simulink model "hydraulic_pilot_dashboard_US"  (R2015b)
settings: Solver=ode23t  StartTime=0.0  StopTime=1500  RelTol=1e-3
undefined symbols (not defined in the file): X, Y, Z
libraries: sm_lib x295, fl_lib x24, nesl_utility x13, sh_lib x5, simulink x1
(part 1 of 7)
settings Model: Creator=Ivan  LastModifiedBy=Ivan
settings DataIOCC: SaveFormat=Array
settings DebuggingCC: UnderspecifiedInitializationDetection=Classic  MergeDetectMultiDrivingBlocksExec=none  SolverPrmCheckMsg=warning  StateNameClashWarn=warning
settings HardwareCC: ProdBitPerPointer=32  ProdLargestAtomicFloat=None  ProdIntDivRoundTo=Undefined  ProdEndianess=Unspecified  ProdWordSize=32  ProdHWDeviceType=32-bit Generic
settings GRTTargetCC: GeneratePreprocessorConditionals=Disable all
settings ConfigComp: CovModelRefEnable=Off
settings SimscapeCC: SimscapeLogType=all  SimscapeLogLimitData=off
settings ExplorerConfigSet: InternalSimMechanicsExplorerSettings="<ExplorerConfiguration><canonicalview>default</canonicalview><AnimationSetting><BasePlaybackSpeed>1.0</BasePlaybackSpeed><PlaybackSpeedFactor>16.0</PlaybackSpeedFactor></AnimationSetting><TilePanel><TileInfo><Tiles Columns=\"2\" Count=\"4\" Rows=\"2\"><Column Left=\"2\" Weight=\"0.5\"/><Column Left=\"554\" Weight=\"0.5\"/><Column Left=\"1106\"/><Row Top=\"2\" Weight=\"0.4992\"/><Row Top=\"320\" Weight=\"0.5008\"/><Row Top=\"639\"/><Tile Height=\"1\" Width=\"1\" X=\"0\" Y=\"0\"/><Tile Height=\"1\" Width=\"1\" X=\"0\" Y=\"1\"/><Tile Height=\"1\" Width=\"1\" X=\"1\" Y=\"0\"/><Tile Height=\"1\" Width=\"1\" X=\"1\" Y=\"1\"/></Tiles></TileInfo><SceneInfo><SceneViewer><BGColor><R>0.60000002384185791</R><G>0.60000002384185791</G><B>0.60000002384185791</B></BGColor><Camera><Position><X>-1.4545420789578025</X><Y>-0.47703526853152423</Y><Z>1.053292472596125</Z></Position><Center><X>-1.0755331343287176</X><Y>0.65681441625729753</Y><Z>0.33046154790126991</Z></Center><Up><X>0.31799715127972389</X><Y>0.43179203595848165</Y><Z>0.84405772874893448</Z></Up><Left>-0.52137946486473086</Left><Right>0.52137946486473086</Right><Bottom>-0.12744375988841058</Bottom><Top>0.12744375988841058</Top></Camera></SceneViewer><SceneViewer><BGColor><R>0.60000002384185791</R><G>0.60000002384185791</G><B>0.60000002384185791</B></BGColor><Camera><Position><X>-1.097124655307177</X><Y>0.60879350298107193</Y><Z>1.6773847746848054</Z></Position><Center><X>-1.097124655307177</X><Y>0.60879350298107193</Y><Z>0.3230140209197998</Z></Center><Up><X>0</X><Y>1</Y><Z>-0</Z></Up><Left>-0.52137946486473086</Left><Right>0.52137946486473086</Right><Bottom>-0.19162502065300943</Bottom><Top>0.19162502065300943</Top></Camera></SceneViewer><SceneViewer><BGColor><R>0.60000002384185791</R><G>0.60000002384185791</G><B>0.60000002384185791</B></BGColor><Camera><Position><X>-1.839713975613805</X><Y>1.4497817237667032</Y><Z>1.0667372871108483</Z></Position><Center><X>-1.0007040048852538</X><Y>0.55541256489420043</Y><Z>0.26430212739881542</Z></Center><Up><X>0.29701754457873719</X><Y>-0.46808723288325788</Y><Z>0.83227094183571793</Z></Up><Left>-0.47525307471029621</Left><Right>0.47525307471029621</Right><Bottom>-0.31607583672115108</Bottom><Top>0.31607583672115108</Top></Camera></SceneViewer><SceneViewer><BGColor><R>0.60000002384185791</R><G>0.60000002384185791</G><B>0.60000002384185791</B></BGColor><Camera><Position><X>-0.30663977538297038</X><Y>-0.17371608341982503</Y><Z>1.1012231263046517</Z></Position><Center><X>-1.0848488807678223</X><Y>0.60449302196502686</Y><Z>0.3230140209197998</Z></Center><Up><X>-0.40824829046386307</X><Y>0.40824829046386307</Y><Z>0.81649658092772615</Z></Up><Left>-0.50417031347751617</Left><Right>0.50417031347751617</Right><Bottom>-0.39514026045799255</Bottom><Top>0.39514026045799255</Top></Camera></SceneViewer></SceneInfo></TilePanel></ExplorerConfiguration>"

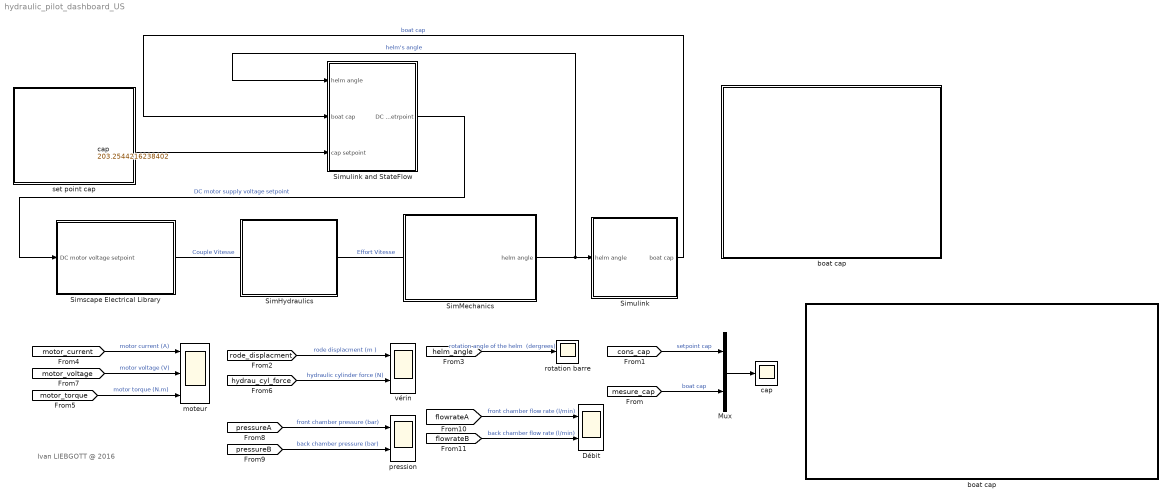
== system hydraulic_pilot_dashboard_US ==
  note: Ivan LIEBGOTT @ 2016
  " moteur" : Scope  NumInputPorts=3
  Débit : Scope  NumInputPorts=2
  Mux : Mux  Inputs=2
  SimHydraulics : Subsystem
      mask Display: image('groupe_hydraulique.jpg')
  SimMechanics : Subsystem
      mask Display: image('pilote_simmechanics.jpg')
  "Simscape Electrical Library " : Subsystem
      mask Display: image('moteur_cc_pilote.jpg')
  Simulink : Subsystem
      mask Display: image('bateau.jpg')
  Simulink and StateFlow : Subsystem
      mask Display: image('AP16_FRONT.jpg')
  boat cap : Subsystem  DialogController=hmiCreateDDGDialog  IsWebBlock=on  mask(MathWorksWebBlock){webBlockId=e22fa1aa-ddbe-4e38-8835-48dbfeb78bab, webBlockType=sdiscope, ShowInitialText=on, HMISrcModelName=hydraulic_pilot_dashboard_US}
      mask prompts: webBlockId "WebBlock Id"; webBlockType "WebBlock Type"; HMISrcModelName "Source Model"
      mask Help: helpview([docroot '/mapfiles/simulink.map'], 'hmi_scope')
      mask Display:
      | if strcmp(get_param(bdroot(gcb),'BlockDiagramType'), 'library')
      |     image([(matlabroot) '/toolbox/simulink/hmi/icons/DashboardScope.png']);
      | end
  "boat cap " : Subsystem  DialogController=hmiCreateDDGDialog  IsWebBlock=on  mask(MathWorksWebBlock){webBlockId=00e2b6f1-632d-4b1a-952e-7d57ffc56f45, webBlockType=circulargauge, ShowInLibBrowser=on, ShowInitialText=on, HMISrcModelName=hydraulic_pilot_dashboard_US}
      mask prompts: webBlockId "WebBlock Id"; webBlockType "WebBlock Type"; HMISrcModelName "Source Model"
      mask Help: helpview([docroot '/mapfiles/simulink.map'], 'hmi_gauge')
      mask Display:
      | if strcmp(get_param(bdroot(gcb),'BlockDiagramType'), 'library')
      |     image([(matlabroot) '/toolbox/simulink/hmi/icons/CircularGauge.png']);
      | end
  cap : Constant  Value=203.2544216238402
  "cap " : Scope
  pression : Scope  NumInputPorts=2
  rotation barre : Scope
  set point cap : Subsystem  DialogController=hmiCreateDDGDialog  IsWebBlock=on  mask(MathWorksWebBlock){webBlockId=deb2e274-1bba-45a5-ab0e-2b4103336ddf, webBlockType=continuousknob, ShowInLibBrowser=on, ShowInitialText=on, HMISrcModelName=hydraulic_pilot_dashboard_US}
      mask prompts: webBlockId "WebBlock Id"; webBlockType "WebBlock Type"; HMISrcModelName "Source Model"
      mask Help: helpview([docroot '/mapfiles/simulink.map'], 'hmi_knob')
      mask Display:
      | if strcmp(get_param(bdroot(gcb),'BlockDiagramType'), 'library')
      |     image([(matlabroot) '/toolbox/simulink/hmi/icons/ContinuousKnob.png']);
      | end
  vérin : Scope  NumInputPorts=2
  wires:
  SimMechanics/1(helm angle) -> Simulink/1(helm angle), Simulink and StateFlow/1(helm angle)  "helm's angle"
  Mux/1 -> "cap "/1
  [mesure_cap] -> Mux/2  "boat cap"
  [cons_cap] -> Mux/1  "setpoint cap"
  [rode_displacment] -> vérin/1  "rode displacment (m )"
  [helm_angle] -> rotation barre/1  "rotation angle of the helm  (dergrees)"
  [motor_current] -> " moteur"/1  "motor current (A)"
  [motor_torque] -> " moteur"/3  "motor torque (N.m)"
  [hydrau_cyl_force] -> vérin/2  "hydraulic cylinder force (N)"
  cap/1 -> Simulink and StateFlow/3(cap setpoint)
  Simulink/1(boat cap) -> Simulink and StateFlow/2(boat cap)  "boat cap"
  Simulink and StateFlow/1(DC motor voltage setrpoint) -> "Simscape Electrical Library "/1(DC motor voltage setpoint)  "DC motor supply voltage setpoint"
  [motor_voltage] -> " moteur"/2  "motor voltage (V)"
  [pressureA] -> pression/1  "front chamber pressure (bar)"
  [pressureB] -> pression/2  "back chamber pressure (bar)"
  [flowrateA] -> Débit/1  "front chamber flow rate (l/min)"
  [flowrateB] -> Débit/2  "back chamber flow rate (l/min)"
  connections:
  "Simscape Electrical Library "/RConn1 -- SimHydraulics/LConn1  "Couple Vitesse"
  SimHydraulics/RConn1 -- SimMechanics/LConn1  "Effort Vitesse"

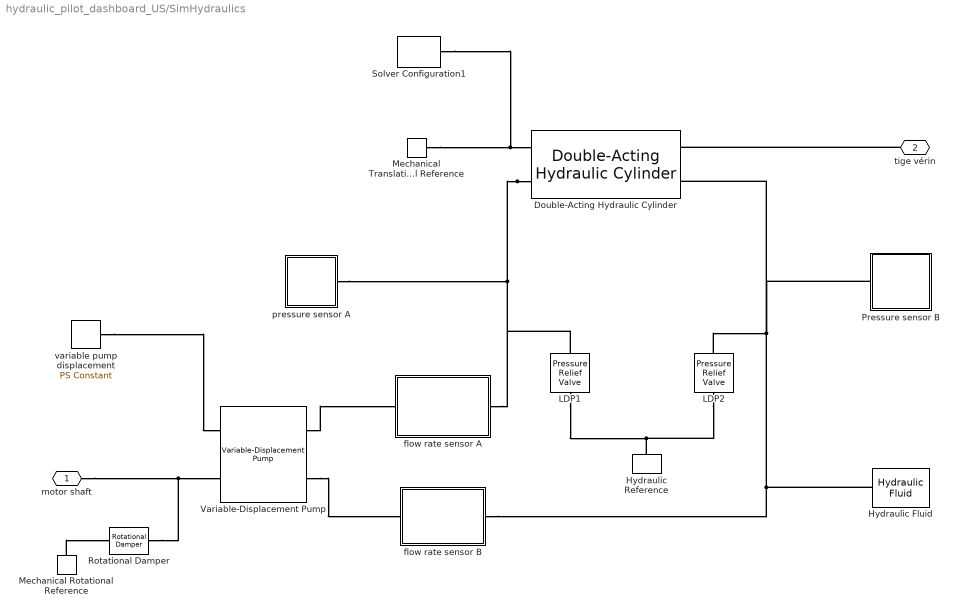
== system hydraulic_pilot_dashboard_US/SimHydraulics ==
  " LDP1" : sh_lib/Valves/Pressure Control Valves/Pressure Relief Valve  area_max=1e-4 m^2  pres_set=10e+6 Pa  reg_range=5e+5 Pa  C_d=0.7  Re_cr=12  A_leak=1e-12 m^2  dynamic=0  tau=0.1 s  area_init=1e-12 m^2  gain=1 m^2/Pa  pr_max=55e5 Pa  f_cr=100 N
  Double-Acting Hydraulic Cylinder : sh_lib/Hydraulic Cylinders/Double-Acting Hydraulic Cylinder  area_A=2e-4 m^2  area_B=2e-4 m^2  stroke=0.3 m  init_pos=0.15 m  dead_vol_A=1e-4 m^3  dead_vol_B=1e-4 m^3  init_pressure_A=0 Pa  init_pressure_B=0 Pa  k_sh=1.4  stiff=1e+6 N/m  D=150 N/(m/s)  or=1  or_sign=1
  Hydraulic Fluid : sh_lib/Hydraulic Utilities/Hydraulic Fluid  DataSource=1  SelFluid=1  SysTemp=60 c  TrapAir=0.005  ViscDerFactor=1  range_error=2
  Hydraulic Reference : fl_lib/Hydraulic/Hydraulic Elements/Hydraulic Reference
  LDP2 : sh_lib/Valves/Pressure Control Valves/Pressure Relief Valve  area_max=1e-4 m^2  pres_set=10e+6 Pa  reg_range=5e+5 Pa  C_d=0.7  Re_cr=12  A_leak=1e-12 m^2  dynamic=0  tau=0.1 s  area_init=1e-12 m^2  gain=1 m^2/Pa  pr_max=55e5 Pa  f_cr=100 N
  Mechanical Rotational Reference : fl_lib/Mechanical/Rotational Elements/Mechanical Rotational Reference
  Mechanical Translational Reference : fl_lib/Mechanical/Translational Elements/Mechanical Translational Reference
  Pressure sensor B : Subsystem
      mask Display: image('manometre.jpg')
  Rotational Damper : fl_lib/Mechanical/Rotational Elements/Rotational Damper  D=0.006 N*m/(rad/s)  w_specify=off  w_priority=None  w=0 rad/s  t_specify=off  t_priority=None  t=0 N*m
  Solver Configuration1 : nesl_utility/Solver Configuration  PhysicalDomain=network_engine_domain  SubClassName=solver  LeftPortType=input  RightPortType=generic  Accelerate=off  Tones=[]  Harmonics=[]  SimulateNoise=off  Profile=off  UseLocalSampling=off  EnableSwitchedLinearOptims=on  FrequencyDomain=off  UseCCode=off  RelTol=0.001  AbsTol=1e-06  MinStep=1e-09  ToWorkspace=off  RevertToSquareIcSolve=off  NumHomotopyIterations=100  PhasorMode=off  PhasorModeNumHarmonics=1  DoDC=off  ResidualTolerance=1e-09  UseLocalSolver=off  LocalSolverChoice=NE_BACKWARD_EULER_ADVANCER  LocalSolverSampleTime=0.001  DoFixedCost=off  MaxNonlinIter=3  MaxModeIter=2  LinearAlgebra=Sparse  DelaysMemoryBudget=1024  AutomaticFiltering=on  FilteringTimeConstant=0.001
  Variable-Displacement Pump : sh_lib/Pumps and Motors/Variable-Displacement Pump  mdl_type=1  D_max=1.77e-7 m^3/rad  stroke_max=1 m  displ_tab=[ -5e-6 -3e-6 0 3e-6 5e-6 ] m^3/rad  cntrl_mem_tab=[ -0.0075 -0.0025 0 0.0025 0.0075 ] m  interp_method=1  extrap_method=1  efficiency_vol=0.85  efficiency_tot=0.75  pr_nominal=1e+8 Pa  w_nominal=188 rad/s  visc_nominal=18 cSt  dens_nominal=900 kg/m^3  k_leak=1e-11 m^3/s/Pa  efficiency_mech=0.7
  flow rate sensor A : Subsystem
      mask Display: image('debimetre.jpg')
  flow rate sensor B : Subsystem
      mask Display: image('debimetre.jpg')
  pressure sensor A : Subsystem
      mask Display: image('manometre.jpg')
  variable pump displacement : fl_lib/Physical Signals/Sources/PS Constant  constant=0.4
  motor shaft : PMIOPort  Port=1  Side=Left
  tige vérin : PMIOPort  Port=2  Side=Right
  connections:
  motor shaft/RConn1 -- Rotational Damper/RConn1 -- Variable-Displacement Pump/LConn2
  variable pump displacement/RConn1 -- Variable-Displacement Pump/LConn1
  tige vérin/RConn1 -- Double-Acting Hydraulic Cylinder/RConn1
  Mechanical Translational Reference/LConn1 -- Solver Configuration1/RConn1 -- Double-Acting Hydraulic Cylinder/LConn1
  Hydraulic Fluid/RConn1 -- flow rate sensor B/RConn1 -- Pressure sensor B/LConn1 -- Double-Acting Hydraulic Cylinder/RConn2 -- LDP2/LConn1
  Hydraulic Reference/LConn1 -- " LDP1"/RConn1 -- LDP2/RConn1
  Mechanical Rotational Reference/LConn1 -- Rotational Damper/LConn1
  Double-Acting Hydraulic Cylinder/LConn2 -- flow rate sensor A/RConn1 -- " LDP1"/LConn1 -- pressure sensor A/RConn1
  Variable-Displacement Pump/RConn1 -- flow rate sensor A/LConn1
  Variable-Displacement Pump/RConn2 -- flow rate sensor B/LConn1

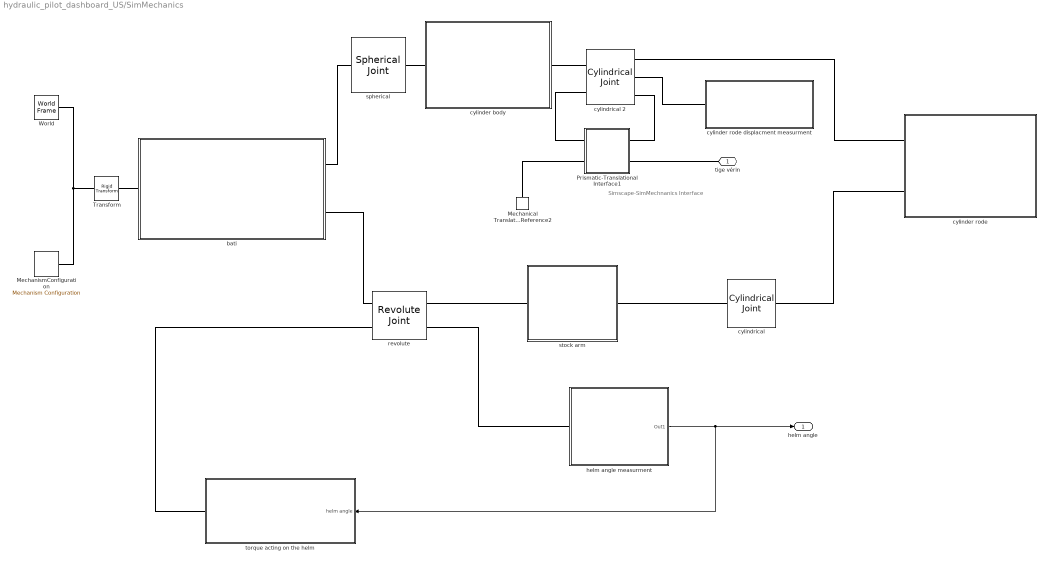
== system hydraulic_pilot_dashboard_US/SimMechanics ==
  note: Simscape-SimMechnanics
      |  Interface
  Mechanical Translational Reference2 : fl_lib/Mechanical/Translational Elements/Mechanical Translational Reference
  MechanismConfiguration : sm_lib/Utilities/Mechanism Configuration  UniformGravity=Constant  GravityVector=[0 0 -9.81]  GravityUnits=m/s^2  LinearizationDelta=0.001  BlockFunction=simmechanics.library.utilities.mechanism_configuration
  Prismatic-Translational Interface1 : Subsystem
  Transform : sm_lib/Frames and Transforms/Rigid Transform  TranslationMethod=Cartesian  TranslationLengthUnit=mm  TranslationStandardAxis=+Z  TranslationStandardOffset=0  TranslationCartesianOffset=[-854.29700000000003 517.99300000000005 336.38900000000001]  TranslationROffset=0  TranslationROffsetUnits=m  TranslationZOffset=0  TranslationZOffsetUnits=m  TranslationThetaOffset=0  TranslationThetaOffsetUnits=deg  RotationMethod=None  RotationAngleUnits=deg  RotationStandardAxis=+Z  RotationAngle=0  RotationArbitraryAxis=[0 0 1]  FollAlignAxisA=+X  BaseAlignAxisA=+Y  FollAlignAxisB=+Y  BaseAlignAxisB=+Z  RotationSequenceAxes=FollowerAxes  RotationSequence=XYX  RotationSequenceAngles=[0 0 0]  RotationSequenceAnglesUnits=deg  RotationMatrix=[1 0 0; 0 1 0; 0 0 1]  BlockFunction=simmechanics.library.frames_transforms.rigid_transform
  World : sm_lib/Frames and Transforms/World Frame  BlockFunction=simmechanics.library.frames_transforms.world_frame
  bati : Subsystem
      mask Display: image('bati1.jpg')
  cylinder body : Subsystem
      mask Display: image('cylindre.jpg')
  cylinder rode : Subsystem
      mask Display: image('tige1.jpg')
  cylinder rode displacment measurment : Subsystem
      mask Display: image('potentiometrelineaire.jpg')
  cylindrical : sm_lib/Joints/Cylindrical Joint  SenseConstraintForce=off  SenseConstraintForceX=off  SenseConstraintForceY=off  SenseConstraintForceZ=off  SenseConstraintTorque=off  SenseConstraintTorqueX=off  SenseConstraintTorqueY=off  SenseConstraintTorqueZ=off  SenseTotalForce=off  SenseTotalForceX=off  SenseTotalForceY=off  SenseTotalForceZ=off  SenseTotalTorque=off  SenseTotalTorqueX=off  SenseTotalTorqueY=off  SenseTotalTorqueZ=off  CompositeWrenchDir=FollowerOnBase  CompositeWrenchFrame=BaseFrame  PzEquilibriumPosition=0  PzEquilibriumPositionUnits=m  PzSpringStiffness=0  PzSpringStiffnessUnits=N/m  PzDampingCoefficient=0  PzDampingCoefficientUnits=s*N/m  PzTorqueActuationMode=NoTorque  PzMotionActuationMode=ComputedMotion  PzSensePosition=off  PzSenseVelocity=off  PzSenseAcceleration=off  PzSenseTorqueForce=off  PzPositionTargetSpecify=on  PzPositionTargetPriority=Low  PzPositionTargetValue=0  PzPositionTargetValueUnits=m  PzVelocityTargetSpecify=off  PzVelocityTargetPriority=High  PzVelocityTargetValue=0  PzVelocityTargetValueUnits=m/s  RzEquilibriumPosition=0  RzEquilibriumPositionUnits=rad  RzSpringStiffness=0  RzSpringStiffnessUnits=m*N/rad  RzDampingCoefficient=0  RzDampingCoefficientUnits=m*s*N/rad  RzTorqueActuationMode=NoTorque  RzMotionActuationMode=ComputedMotion  RzSensePosition=off  RzSenseVelocity=off  RzSenseAcceleration=off  RzSenseTorqueForce=off  RzPositionTargetSpecify=on  RzPositionTargetPriority=Low  RzPositionTargetValue=88.917590363493801  RzPositionTargetValueUnits=deg  RzVelocityTargetSpecify=off  RzVelocityTargetPriority=High  RzVelocityTargetValue=0  RzVelocityTargetValueUnits=deg/s  BlockFunction=simmechanics.library.joints.cylindrical_joint
  cylindrical 2 : sm_lib/Joints/Cylindrical Joint  SenseConstraintForce=off  SenseConstraintForceX=off  SenseConstraintForceY=off  SenseConstraintForceZ=off  SenseConstraintTorque=off  SenseConstraintTorqueX=off  SenseConstraintTorqueY=off  SenseConstraintTorqueZ=off  SenseTotalForce=off  SenseTotalForceX=off  SenseTotalForceY=off  SenseTotalForceZ=off  SenseTotalTorque=off  SenseTotalTorqueX=off  SenseTotalTorqueY=off  SenseTotalTorqueZ=off  CompositeWrenchDir=FollowerOnBase  CompositeWrenchFrame=BaseFrame  PzEquilibriumPosition=0  PzEquilibriumPositionUnits=m  PzSpringStiffness=0  PzSpringStiffnessUnits=N/m  PzDampingCoefficient=0  PzDampingCoefficientUnits=s*N/m  PzTorqueActuationMode=InputTorque  PzMotionActuationMode=ComputedMotion  PzSensePosition=on  PzSenseVelocity=on  PzSenseAcceleration=off  PzSenseTorqueForce=off  PzPositionTargetSpecify=on  PzPositionTargetPriority=Low  PzPositionTargetValue=0  PzPositionTargetValueUnits=m  PzVelocityTargetSpecify=off  PzVelocityTargetPriority=High  PzVelocityTargetValue=0  PzVelocityTargetValueUnits=m/s  RzEquilibriumPosition=0  RzEquilibriumPositionUnits=rad  RzSpringStiffness=0  RzSpringStiffnessUnits=m*N/rad  RzDampingCoefficient=1  RzDampingCoefficientUnits=m*s*N/rad  RzTorqueActuationMode=NoTorque  RzMotionActuationMode=ComputedMotion  RzSensePosition=off  RzSenseVelocity=off  RzSenseAcceleration=off  RzSenseTorqueForce=off  RzPositionTargetSpecify=on  RzPositionTargetPriority=Low  RzPositionTargetValue=-151.66852375213551  RzPositionTargetValueUnits=deg  RzVelocityTargetSpecify=off  RzVelocityTargetPriority=High  RzVelocityTargetValue=0  RzVelocityTargetValueUnits=deg/s  BlockFunction=simmechanics.library.joints.cylindrical_joint
  helm angle measurment : Subsystem
      mask Display: image('potentiometreangle.jpg')
  revolute : sm_lib/Joints/Revolute Joint  SenseConstraintForce=off  SenseConstraintForceX=off  SenseConstraintForceY=off  SenseConstraintForceZ=off  SenseConstraintTorque=off  SenseConstraintTorqueX=off  SenseConstraintTorqueY=off  SenseConstraintTorqueZ=off  SenseTotalForce=off  SenseTotalForceX=off  SenseTotalForceY=off  SenseTotalForceZ=off  SenseTotalTorque=off  SenseTotalTorqueX=off  SenseTotalTorqueY=off  SenseTotalTorqueZ=off  CompositeWrenchDir=FollowerOnBase  CompositeWrenchFrame=BaseFrame  EquilibriumPosition=0  EquilibriumPositionUnits=rad  SpringStiffness=0  SpringStiffnessUnits=m*N/rad  DampingCoefficient=0  DampingCoefficientUnits=m*s*N/rad  TorqueActuationMode=InputTorque  MotionActuationMode=ComputedMotion  SensePosition=on  SenseVelocity=off  SenseAcceleration=off  SenseTorqueForce=off  PositionTargetSpecify=on  PositionTargetPriority=Low  PositionTargetValue=91.342079820133691  PositionTargetValueUnits=deg  VelocityTargetSpecify=off  VelocityTargetPriority=High  VelocityTargetValue=0  VelocityTargetValueUnits=deg/s  BlockFunction=simmechanics.library.joints.revolute_joint
  spherical : sm_lib/Joints/Spherical Joint  SenseConstraintForce=off  SenseConstraintForceX=off  SenseConstraintForceY=off  SenseConstraintForceZ=off  SenseConstraintTorque=off  SenseConstraintTorqueX=off  SenseConstraintTorqueY=off  SenseConstraintTorqueZ=off  SenseTotalForce=off  SenseTotalForceX=off  SenseTotalForceY=off  SenseTotalForceZ=off  SenseTotalTorque=off  SenseTotalTorqueX=off  SenseTotalTorqueY=off  SenseTotalTorqueZ=off  CompositeWrenchDir=FollowerOnBase  CompositeWrenchFrame=BaseFrame  DefPosRotationMethod=None  DefPosRotationAngleUnits=deg  DefPosRotationStandardAxis=+Z  DefPosRotationAngle=0  DefPosRotationArbitraryAxis=[0 0 1]  DefPosFollAlignAxisA=+X  DefPosBaseAlignAxisA=+Y  DefPosFollAlignAxisB=+Y  DefPosBaseAlignAxisB=+Z  DefPosRotationSequenceAxes=FollowerAxes  DefPosRotationSequence=XYX  DefPosRotationSequenceAngles=[0 0 0]  DefPosRotationSequenceAnglesUnits=deg  DefPosRotationMatrix=[1 0 0; 0 1 0; 0 0 1]  EqPosRotationMethod=None  EqPosRotationAngleUnits=deg  EqPosRotationStandardAxis=+Z  EqPosRotationAngle=0  EqPosRotationArbitraryAxis=[0 0 1]  EqPosFollAlignAxisA=+X  EqPosBaseAlignAxisA=+Y  EqPosFollAlignAxisB=+Y  EqPosBaseAlignAxisB=+Z  EqPosRotationSequenceAxes=FollowerAxes  EqPosRotationSequence=XYX  EqPosRotationSequenceAngles=[0 0 0]  EqPosRotationSequenceAnglesUnits=deg  EqPosRotationMatrix=[1 0 0; 0 1 0; 0 0 1]  SpringStiffness=0  SpringStiffnessUnits=m*N/rad  DampingCoefficient=0  DampingCoefficientUnits=m*s*N/rad  ActuateTorqueX=off  ActuateTorqueY=off  ActuateTorqueZ=off  ActuateTorque=off  TorqueActuationMode=NoTorque  MotionActuationMode=ComputedMotion  ActuationFrame=BaseFrame  SensePosition=off  SenseVelocityX=off  SenseVelocityY=off  SenseVelocityZ=off  SenseVelocity=off  SenseAccelerationX=off  SenseAccelerationY=off  SenseAccelerationZ=off  SenseAcceleration=off  SenseTorqueX=off  SenseTorqueY=off  SenseTorqueZ=off  SenseTorqueForce=off  SensingFrame=FollowerFrame  PositionTargetRotationMethod=None  PositionTargetRotationAngleUnits=deg  PositionTargetRotationStandardAxis=+Z  PositionTargetRotationAngle=0  PositionTargetRotationArbitraryAxis=[0 0 1]  PositionTargetFollAlignAxisA=+X  PositionTargetBaseAlignAxisA=+Y  PositionTargetFollAlignAxisB=+Y  PositionTargetBaseAlignAxisB=+Z  PositionTargetRotationSequenceAxes=FollowerAxes  PositionTargetRotationSequence=XYX  PositionTargetRotationSequenceAngles=[0 0 0]  PositionTargetRotationSequenceAnglesUnits=deg  PositionTargetRotationMatrix=[1 0 0; 0 1 0; 0 0 1]  PositionTargetSpecify=off  PositionTargetPriority=High  VelocityTargetValue=[0 0 0]  VelocityTargetValueUnits=deg/s  VelocityTargetSpecify=off  VelocityTargetPriority=High  VelocityTargetInFollowerFrame=on  BlockFunction=simmechanics.library.joints.spherical_joint
  stock arm : Subsystem
      mask Display: image('meche.jpg')
  torque acting on the helm : Subsystem
  "tige vérin " : PMIOPort  Port=1  Side=Left
  helm angle : Outport
  wires:
  helm angle measurment/1(Out1) -> helm angle/1, torque acting on the helm/1(helm angle)
  connections:
  bati/LConn1 -- Transform/RConn1
  cylinder body/LConn1 -- spherical/RConn1
  bati/RConn1 -- spherical/LConn1
  revolute/RConn1 -- stock arm/LConn1
  revolute/LConn1 -- bati/RConn2
  cylindrical/LConn1 -- stock arm/RConn1
  Transform/LConn1 -- World/RConn1 -- MechanismConfiguration/RConn1
  "tige vérin "/RConn1 -- Prismatic-Translational Interface1/LConn2
  Mechanical Translational Reference2/LConn1 -- Prismatic-Translational Interface1/RConn2
  Prismatic-Translational Interface1/RConn1 -- cylindrical 2/LConn2
  cylindrical 2/RConn3 -- Prismatic-Translational Interface1/LConn1
  cylindrical/RConn1 -- cylinder rode/LConn2
  torque acting on the helm/RConn1 -- revolute/LConn2
  cylinder body/RConn1 -- cylindrical 2/LConn1
  cylindrical 2/RConn1 -- cylinder rode/LConn1
  helm angle measurment/LConn1 -- revolute/RConn2
  cylinder rode displacment measurment/LConn1 -- cylindrical 2/RConn2

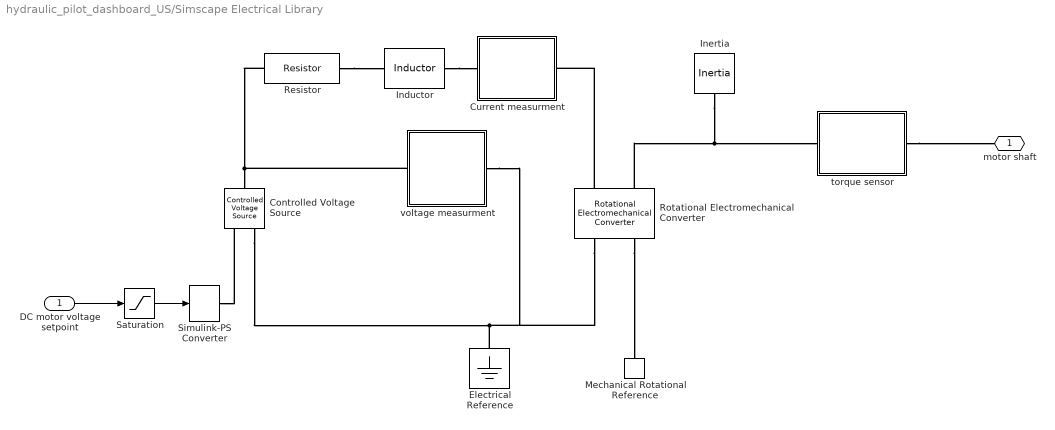
== system hydraulic_pilot_dashboard_US/Simscape Electrical Library  ==
  DC motor voltage setpoint : Inport
  Controlled Voltage Source : fl_lib/Electrical/Electrical Sources/Controlled Voltage Source
  Current measurment : Subsystem
      mask Display: image('ampermetre.jpg')
  Electrical Reference : fl_lib/Electrical/Electrical Elements/Electrical Reference
  Inductor : fl_lib/Electrical/Electrical Elements/Inductor  l=1e-7 H  r=0 Ohm  g=1e-9 1/Ohm  i_specify=off  i_priority=None  i=0 A  v_specify=off  v_priority=None  v=0 V  i_L_specify=on  i_L_priority=High  i_L=0 A
  Inertia : fl_lib/Mechanical/Rotational Elements/Inertia  inertia=0.005 kg*m^2  w_specify=on  w_priority=High  w=0 rad/s  t_specify=off  t_priority=None  t=0 N*m
  Mechanical Rotational Reference : fl_lib/Mechanical/Rotational Elements/Mechanical Rotational Reference
  Resistor : fl_lib/Electrical/Electrical Elements/Resistor  R=0.247 Ohm  i_specify=off  i_priority=None  i=0 A  v_specify=off  v_priority=None  v=0 V
  Rotational Electromechanical Converter : fl_lib/Electrical/Electrical Elements/Rotational Electromechanical Converter  K=0.047 V/(rad/s)  i_specify=off  i_priority=None  i=0 A  v_specify=off  v_priority=None  v=0 V  t_specify=off  t_priority=None  t=0 N*m  w_specify=off  w_priority=None  w=0 rad/s
  Saturation : Saturate  UpperLimit=12  LowerLimit=-12
  Simulink-PS Converter : nesl_utility/Simulink-PS Converter  PhysicalDomain=network_engine_domain  SubClassName=ps_input  LeftPortType=input  RightPortType=output  PseudoPeriodic=off  Frequencies=[]  NoiseDistribution=none  NoiseParameters=[]  Unit=V  AffineConversion=off  InputFiltering=off  SimscapeFilterOrder=1  InputFilterTimeConstant=0.001  UdotUserProvided=1
  torque sensor : Subsystem
      mask Display: image('couplemetre.jpg')
  voltage measurment : Subsystem
      mask Display: image('voltmetre.jpg')
  motor shaft : PMIOPort  Port=1  Side=Right
  wires:
  DC motor voltage setpoint/1 -> Saturation/1
  Saturation/1 -> Simulink-PS Converter/1
  connections:
  Simulink-PS Converter/RConn1 -- Controlled Voltage Source/RConn1
  Rotational Electromechanical Converter/RConn2 -- Mechanical Rotational Reference/LConn1
  Electrical Reference/LConn1 -- Controlled Voltage Source/RConn2 -- voltage measurment/RConn1 -- Rotational Electromechanical Converter/RConn1
  Resistor/LConn1 -- voltage measurment/LConn1 -- Controlled Voltage Source/LConn1
  Resistor/RConn1 -- Inductor/LConn1
  Inductor/RConn1 -- Current measurment/LConn1
  Rotational Electromechanical Converter/LConn1 -- Current measurment/RConn1
  Inertia/LConn1 -- Rotational Electromechanical Converter/LConn2 -- torque sensor/LConn1
  torque sensor/RConn1 -- motor shaft/RConn1

== system hydraulic_pilot_dashboard_US/Simulink ==
  helm angle : Inport
  Integrator : Integrator
  Perturbation : Subsystem
      mask Display: image('vague.jpg')
  Sum : Sum  Inputs=-+|
  Transfer Fcn1 : TransferFcn  Numerator=[0.005]  Denominator=[1 0.1]
  boat cap : Outport
  wires:
  helm angle/1 -> Transfer Fcn1/1
  Integrator/1 -> boat cap/1
  Sum/1 -> Integrator/1
  Transfer Fcn1/1 -> Sum/2
  Perturbation/1(Out1) -> Sum/1

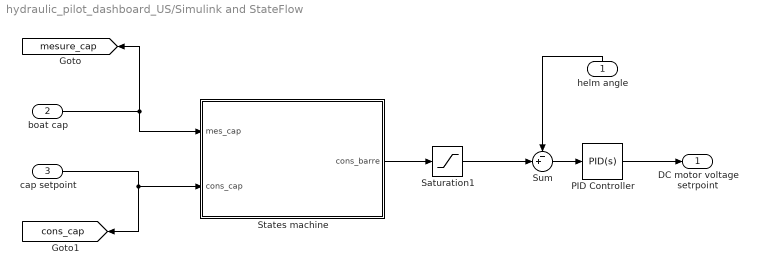
== system hydraulic_pilot_dashboard_US/Simulink and StateFlow ==
  helm angle : Inport
  boat cap : Inport  Port=2
  cap setpoint : Inport  Port=3
  PID Controller : simulink/Continuous/PID Controller  Controller=PID  TimeDomain=Continuous-time  SampleTime=-1  IntegratorMethod=Forward Euler  FilterMethod=Forward Euler  Form=Parallel  UseFilter=on  ControllerParametersSource=internal  P=0.5  I=0.001  D=0  N=100  InitialConditionSource=internal  InitialConditionForIntegrator=0  InitialConditionForFilter=0  ExternalReset=none  LimitOutput=off  UpperSaturationLimit=inf  LowerSaturationLimit=-inf  LinearizeAsGain=on  AntiWindupMode=none  Kb=1  TrackingMode=off  Kt=1  PParamMin=[]  PParamMax=[]  IParamMin=[]  IParamMax=[]  DParamMin=[]  DParamMax=[]  NParamMin=[]  NParamMax=[]  KbParamMin=[]  KbParamMax=[]  KtParamMin=[]  KtParamMax=[]  POutMin=[]  POutMax=[]  IOutMin=[]  IOutMax=[]  DOutMin=[]  DOutMax=[]  NOutMin=[]  NOutMax=[]  KbOutMin=[]  KbOutMax=[]  KtOutMin=[]  KtOutMax=[]  IntegratorOutMin=[]  IntegratorOutMax=[]  FilterOutMin=[]  FilterOutMax=[]  SumOutMin=[]  SumOutMax=[]  SumI1OutMin=[]  SumI1OutMax=[]  SumI2OutMin=[]  SumI2OutMax=[]  SumI3OutMin=[]  SumI3OutMax=[]  SumDOutMin=[]  SumDOutMax=[]  SaturationOutMin=[]  SaturationOutMax=[]  IntegratorContinuousStateAttributes=''  IntegratorStateMustResolveToSignalObject=off  IntegratorRTWStateStorageClass=Auto  FilterContinuousStateAttributes=''  FilterStateMustResolveToSignalObject=off  FilterRTWStateStorageClass=Auto  DifferentiatorICPrevScaledInput=0  DifferentiatorOutMin=[]  DifferentiatorOutMax=[]
  Saturation1 : Saturate  UpperLimit=25  LowerLimit=-25
  States machine : Stateflow chart  TreatAsAtomicUnit=on
  Sum : Sum  Inputs=-+|
  DC motor voltage setrpoint : Outport
  tag scope: cons_cap=global, mesure_cap=global
  wires:
  helm angle/1 -> Sum/1
  cap setpoint/1 -> States machine/2(cons_cap), [cons_cap]
  boat cap/1 -> [mesure_cap], States machine/1(mes_cap)
  Sum/1 -> PID Controller/1
  PID Controller/1 -> DC motor voltage setrpoint/1
  States machine/1(cons_barre) -> Saturation1/1
  Saturation1/1 -> Sum/2

== system hydraulic_pilot_dashboard_US/boat cap ==

== system hydraulic_pilot_dashboard_US/boat cap  ==

== system hydraulic_pilot_dashboard_US/set point cap ==

== system hydraulic_pilot_dashboard_US/SimHydraulics/Pressure sensor B ==
  Hydraulic Pressure Sensor1 : fl_lib/Hydraulic/Hydraulic Sensors/Hydraulic Pressure Sensor
  Hydraulic Reference2 : fl_lib/Hydraulic/Hydraulic Elements/Hydraulic Reference
  PS-Simulink Converter3 : nesl_utility/PS-Simulink Converter  PhysicalDomain=network_engine_domain  SubClassName=ps_output  LeftPortType=input  RightPortType=output  PseudoPeriodic=off  Frequencies=[]  Unit=bar  AffineConversion=off
  Conn1 : PMIOPort  Port=1  Side=Left
  tag scope: pressureB=global
  wires:
  PS-Simulink Converter3/1 -> [pressureB]
  connections:
  Hydraulic Reference2/LConn1 -- Hydraulic Pressure Sensor1/RConn1
  Hydraulic Pressure Sensor1/RConn2 -- PS-Simulink Converter3/LConn1
  Hydraulic Pressure Sensor1/LConn1 -- Conn1/RConn1

== system hydraulic_pilot_dashboard_US/SimHydraulics/flow rate sensor A ==
  Hydraulic Flow Rate Sensor : fl_lib/Hydraulic/Hydraulic Sensors/Hydraulic Flow Rate Sensor
  PS-Simulink Converter4 : nesl_utility/PS-Simulink Converter  PhysicalDomain=network_engine_domain  SubClassName=ps_output  LeftPortType=input  RightPortType=output  PseudoPeriodic=off  Frequencies=[]  Unit=l/min  AffineConversion=off
  Conn1 : PMIOPort  Port=1  Side=Right
  Conn2 : PMIOPort  Port=2  Side=Left
  tag scope: flowrateA=global
  wires:
  PS-Simulink Converter4/1 -> [flowrateA]
  connections:
  Conn2/RConn1 -- Hydraulic Flow Rate Sensor/LConn1
  Hydraulic Flow Rate Sensor/RConn1 -- PS-Simulink Converter4/LConn1
  Hydraulic Flow Rate Sensor/RConn2 -- Conn1/RConn1

== system hydraulic_pilot_dashboard_US/SimHydraulics/flow rate sensor B ==
  Hydraulic Flow Rate Sensor1 : fl_lib/Hydraulic/Hydraulic Sensors/Hydraulic Flow Rate Sensor
  PS-Simulink Converter5 : nesl_utility/PS-Simulink Converter  PhysicalDomain=network_engine_domain  SubClassName=ps_output  LeftPortType=input  RightPortType=output  PseudoPeriodic=off  Frequencies=[]  Unit=l/min  AffineConversion=off
  Conn1 : PMIOPort  Port=1  Side=Right
  Conn2 : PMIOPort  Port=2  Side=Left
  tag scope: flowrateB=global
  wires:
  PS-Simulink Converter5/1 -> [flowrateB]
  connections:
  Conn2/RConn1 -- Hydraulic Flow Rate Sensor1/LConn1
  Hydraulic Flow Rate Sensor1/RConn1 -- PS-Simulink Converter5/LConn1
  Hydraulic Flow Rate Sensor1/RConn2 -- Conn1/RConn1

== system hydraulic_pilot_dashboard_US/SimHydraulics/pressure sensor A ==
  Hydraulic Pressure Sensor : fl_lib/Hydraulic/Hydraulic Sensors/Hydraulic Pressure Sensor
  Hydraulic Reference1 : fl_lib/Hydraulic/Hydraulic Elements/Hydraulic Reference
  PS-Simulink Converter2 : nesl_utility/PS-Simulink Converter  PhysicalDomain=network_engine_domain  SubClassName=ps_output  LeftPortType=input  RightPortType=output  PseudoPeriodic=off  Frequencies=[]  Unit=bar  AffineConversion=off
  Conn1 : PMIOPort  Port=1  Side=Right
  tag scope: pressureA=global
  wires:
  PS-Simulink Converter2/1 -> [pressureA]
  connections:
  Hydraulic Pressure Sensor/LConn1 -- Conn1/RConn1
  PS-Simulink Converter2/LConn1 -- Hydraulic Pressure Sensor/RConn2
  Hydraulic Reference1/LConn1 -- Hydraulic Pressure Sensor/RConn1

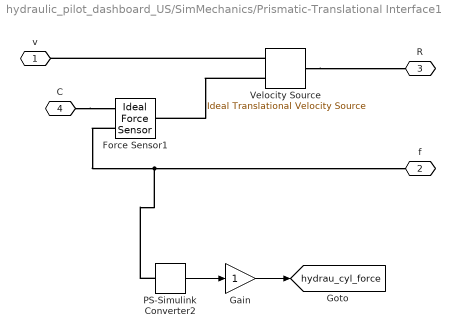
== system hydraulic_pilot_dashboard_US/SimMechanics/Prismatic-Translational Interface1 ==
  Force Sensor1 : fl_lib/Mechanical/Mechanical Sensors/Ideal Force Sensor
  Gain : Gain
  PS-Simulink Converter2 : nesl_utility/PS-Simulink Converter  PhysicalDomain=network_engine_domain  SubClassName=ps_output  LeftPortType=input  RightPortType=output  PseudoPeriodic=off  Frequencies=[]  Unit=N  AffineConversion=off
  Velocity Source : fl_lib/Mechanical/Mechanical Sources/Ideal Translational Velocity Source
  v : PMIOPort  Port=1  Side=Left
  f : PMIOPort  Port=2  Side=Right
  R : PMIOPort  Port=3  Side=Left
  C : PMIOPort  Port=4  Side=Right
  tag scope: hydrau_cyl_force=global
  wires:
  PS-Simulink Converter2/1 -> Gain/1
  Gain/1 -> [hydrau_cyl_force]
  connections:
  Velocity Source/LConn1 -- R/RConn1
  Velocity Source/RConn1 -- v/RConn1
  Force Sensor1/RConn2 -- PS-Simulink Converter2/LConn1 -- f/RConn1
  C/RConn1 -- Force Sensor1/RConn1
  Velocity Source/RConn2 -- Force Sensor1/LConn1

== system hydraulic_pilot_dashboard_US/SimMechanics/bati ==
  AP_Cadre_2_RIGID : Subsystem
  AP_Platine_2_RIGID : Subsystem
  ReferenceFrame : sm_lib/Frames and Transforms/Reference Frame  BlockFunction=simmechanics.library.frames_transforms.reference_frame
  Transform : sm_lib/Frames and Transforms/Rigid Transform  TranslationMethod=Cartesian  TranslationLengthUnit=mm  TranslationStandardAxis=+Z  TranslationStandardOffset=0  TranslationCartesianOffset=[0 -3.5527136788005009e-15 26.61639999999997]  TranslationROffset=0  TranslationROffsetUnits=m  TranslationZOffset=0  TranslationZOffsetUnits=m  TranslationThetaOffset=0  TranslationThetaOffsetUnits=deg  RotationMethod=ArbitraryAxis  RotationAngleUnits=rad  RotationStandardAxis=+Z  RotationAngle=5.5511151231257827e-17  RotationArbitraryAxis=[-0 -1 0]  FollAlignAxisA=+X  BaseAlignAxisA=+Y  FollAlignAxisB=+Y  BaseAlignAxisB=+Z  RotationSequenceAxes=FollowerAxes  RotationSequence=XYX  RotationSequenceAngles=[0 0 0]  RotationSequenceAnglesUnits=deg  RotationMatrix=[1 0 0; 0 1 0; 0 0 1]  BlockFunction=simmechanics.library.frames_transforms.rigid_transform
  Transform1 : sm_lib/Frames and Transforms/Rigid Transform  TranslationMethod=Cartesian  TranslationLengthUnit=mm  TranslationStandardAxis=+Z  TranslationStandardOffset=0  TranslationCartesianOffset=[-593.50000000000011 155 69]  TranslationROffset=0  TranslationROffsetUnits=m  TranslationZOffset=0  TranslationZOffsetUnits=m  TranslationThetaOffset=0  TranslationThetaOffsetUnits=deg  RotationMethod=ArbitraryAxis  RotationAngleUnits=rad  RotationStandardAxis=+Z  RotationAngle=0  RotationArbitraryAxis=[0 0 0]  FollAlignAxisA=+X  BaseAlignAxisA=+Y  FollAlignAxisB=+Y  BaseAlignAxisB=+Z  RotationSequenceAxes=FollowerAxes  RotationSequence=XYX  RotationSequenceAngles=[0 0 0]  RotationSequenceAnglesUnits=deg  RotationMatrix=[1 0 0; 0 1 0; 0 0 1]  BlockFunction=simmechanics.library.frames_transforms.rigid_transform
  F2 : PMIOPort  Port=1  Side=Left
  F1 : PMIOPort  Port=2  Side=Right
  F : PMIOPort  Port=3  Side=Right
  connections:
  AP_Platine_2_RIGID/RConn1 -- AP_Cadre_2_RIGID/RConn1 -- Transform/LConn1 -- Transform1/LConn1 -- F2/RConn1 -- ReferenceFrame/RConn1
  Transform/RConn1 -- F/RConn1
  Transform1/RConn1 -- F1/RConn1
